simulink model "harness"  (R2020b)
settings: Solver=FixedStepDiscrete  StartTime=0.0  StopTime=inf  FixedStep=0.000001  RelTol=1e-3  EnableMultiTasking=on
settings Model: SILPILModeSetting=veronly  EnablePacing=on  PacingRate=0.890000  ExtModeTrigDuration=2  Creator=GUO HUI  LastModifiedBy=GUO HUI
settings OptimizationCC: EnhancedBackFolding=on  PassReuseOutputArgsAs=Individual arguments  MaxStackSize=64  OptimizeBlockOrder=speed  DifferentSizesBufferReuse=on  OptimizationCustomize=off  EfficientTunableParamExpr=on
settings DebuggingCC: ParameterTunabilityLossMsg=error
settings HardwareCC: ProdBitPerInt=16  ProdBitPerPointer=16  ProdBitPerSizeT=16  ProdBitPerPtrDiffT=16  ProdLargestAtomicFloat=None  ProdWordSize=8  ProdHWDeviceType=Atmel->AVR
settings SFSimCC: MATLABDynamicMemAlloc=off
settings RTWCC: Description=Embedded Coder  SystemTargetFile=ert.tlc  HardwareBoard=Arduino Uno  GenCodeOnly=on  TemplateMakefile=ert_default_tmf  GenerateReport=on  Toolchain=Arduino AVR  BuildConfiguration=Faster Runs  IncludeHyperlinkInReport=on  LaunchReport=on  GenerateTraceInfo=on  GenerateCodeMetricsReport=on
settings CodeAppCC: ForceParamTrailComments=on  IgnoreCustomStorageClasses=off  OperatorAnnotations=on  SimulinkDataObjDesc=on  SFDataObjDesc=on  InsertBlockDesc=on
settings ERTTargetCC: CodeInterfacePackaging=Reusable function  SupportContinuousTime=on  SupportVariableSizeSignals=on  ExtModeStaticAllocSize=250  ERTFilePackagingFormat=Compact
settings ConfigComp: CovScope=Subsystem  CovEnableCumulative=off  CovSaveSingleToWorkspaceVar=on  CovExternalEMLEnable=off  CovSFcnEnable=off

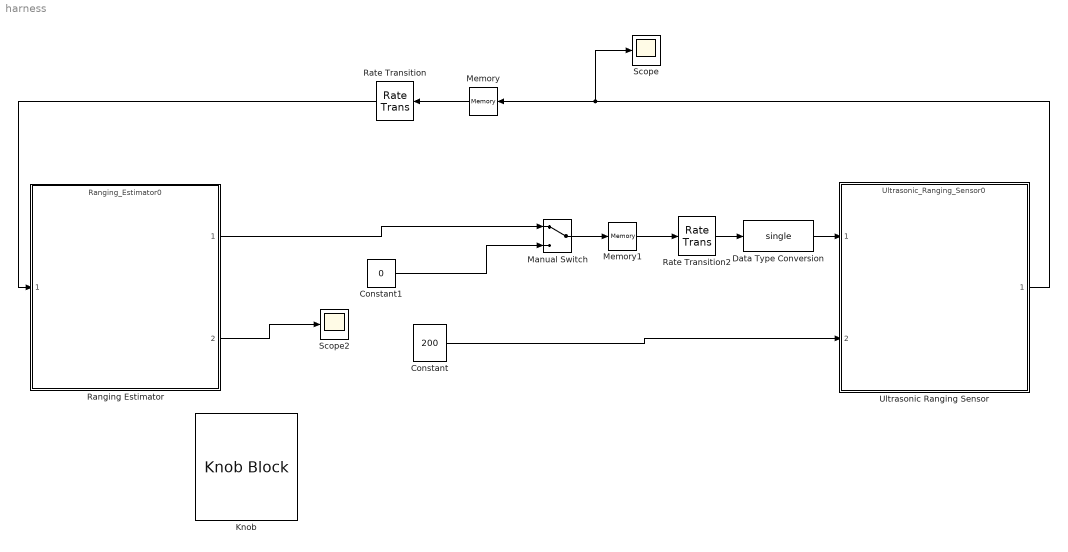
== system harness ==
  Constant : Constant  Value=200
  Constant1 : Constant  Value=0
  Data Type Conversion : DataTypeConversion  OutDataTypeStr=single  LockScale=on
  Knob : KnobBlock
  Manual Switch : ManualSwitch
  Memory : Memory
  Memory1 : Memory
  Ranging Estimator : ModelReference  ModelNameDialog=Ranging_Estimator0  SimulationMode=Normal  ModelReferenceVersion=1.42
  Rate Transition : RateTransition
  Rate Transition2 : RateTransition
  Scope : Scope
  Scope2 : Scope
  Ultrasonic Ranging Sensor : ModelReference  ModelNameDialog=Ultrasonic_Ranging_Sensor0  SimulationMode=Normal  ModelReferenceVersion=1.7
  wires:
  Constant1/1 -> Manual Switch/2
  Ultrasonic Ranging Sensor/1 -> Scope/1, Memory/1
  Memory/1 -> Rate Transition/1
  Rate Transition/1 -> Ranging Estimator/1
  Manual Switch/1 -> Memory1/1
  Memory1/1 -> Rate Transition2/1
  Rate Transition2/1 -> Data Type Conversion/1
  Ranging Estimator/1 -> Manual Switch/1
  Ranging Estimator/2 -> Scope2/1
  Constant/1 -> Ultrasonic Ranging Sensor/2
  Data Type Conversion/1 -> Ultrasonic Ranging Sensor/1
